simulink model "srial_multipleinput"  (R2021b)
settings: Solver=FixedStepAuto  StartTime=0.0  StopTime=inf  FixedStep=0.5  RelTol=1e-3
libraries: instrumentseriallib x3
settings Model: Creator=maral  LastModifiedBy=maral

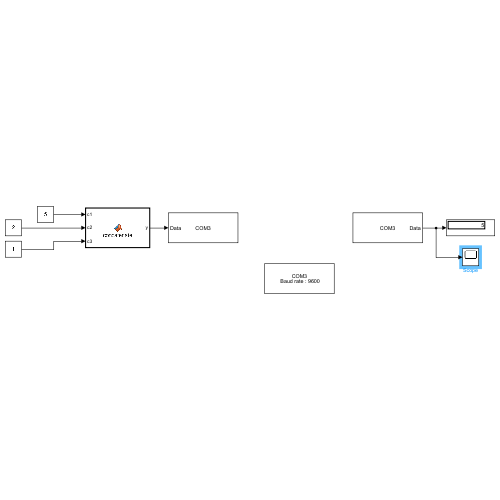
[thumbnail: Simulink's stored preview of the top-level diagram]
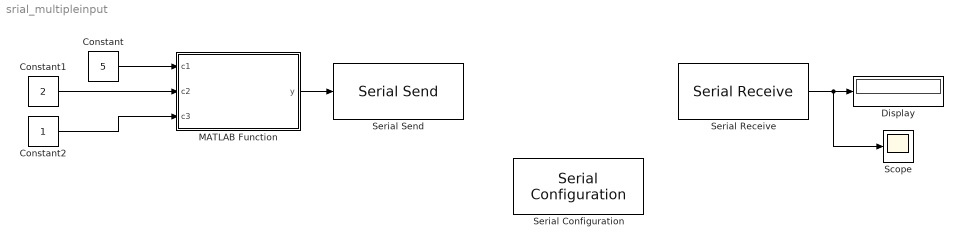
== system srial_multipleinput ==
  Constant : Constant  Value=5  OutDataTypeStr=int8
  Constant1 : Constant  Value=2  OutDataTypeStr=int8
  Constant2 : Constant  OutDataTypeStr=int8
  Display : Display
  MATLAB Function : MATLAB Function  TreatAsAtomicUnit=on
  Scope : Scope
  Serial Configuration : instrumentseriallib/Serial Configuration  Priority=-200000  Port=COM3  ComPort=COM3  BaudRate=9600  DataBits=8  Parity=none  StopBits=1  ByteOrder=little-endian  FlowControl=none  Timeout=10  SimulateUsing=Interpreted execution  BlockInModel=on
  Serial Receive : instrumentseriallib/Serial Receive  Priority=1  Port=COM3  ComPort=COM3  DataType=uint8  SaveDataType=uint8  ToggleHeader=off  Header=[]  ToggleTerminator=off  Terminator=<none>  CustomTerminator=[]  ToggleDataSize=on  DataSize=[1 1]  EnableBlockingMode=on  ActionDataUnavailable=Output last received value  ActionWhenDataUnavailable=Output last received value  CustomValue=0  SampleTime=-1  SimulateUsing=Interpreted execution  BlockInModel=on
  Serial Send : instrumentseriallib/Serial Send  Priority=1  Port=COM3  ComPort=COM3  Header=[]  Terminator=<none>  CustomTerminator=[]  EnableBlockingMode=on  SimulateUsing=Interpreted execution  BlockInModel=on
  wires:
  Serial Receive/1 -> Scope/1, Display/1
  MATLAB Function/1(y) -> Serial Send/1
  Constant/1 -> MATLAB Function/1(c1)
  Constant1/1 -> MATLAB Function/2(c2)
  Constant2/1 -> MATLAB Function/3(c3)

== matlab function srial_multipleinput/MATLAB Function ==
  data: c1 input; y output; c2 input; c3 input
function y = concatenate(c1, c2, c3)
y = [c1 c2 c3];
end
